simulink model "mariner_sim"  (R2018b)
(part 16 of 22)

  "IW{3,2}(6,:)'" : Constant  Value=[0.341232504422672555666196103629772551357746124267578125;-0.22407651602017242264963670095312409102916717529296875;-0.149532198205526156709055385363171808421611785888671875;-0.20169871649001336333384415411273948848247528076171875;0.1757399362782041396524590481931227259337902069091796875;0.05540417170915674927034189067853731103241443634033203125;0.0032609465010274645523080661035919547430239617824554443359375;-0.22300988569188906485152301684138365089893341064453125;-0.22795024991608858755398614448495209217071533203125;0.0919947464537682335627977181502501480281352996826171875;0.07236540787619029357902178389849723316729068756103515625;-0.019836013133734016478104678071758826263248920440673828125;-0.29188822221009502744237806837190873920917510986328125;0.30454637581194088369329620036296546459197998046875;-0.01535199508936785535440083805269750882871448993682861328125;0.36874333544784054783605142802116461098194122314453125;-0.361608618282780069908000086797983385622501373291015625;-0.30980629966419837018065663869492709636688232421875;-0.310442442961680609148089615700882859528064727783203125;0.006138782561133275007814180668219705694355070590972900390625;-0.1582495940895217445554266078033833764493465423583984375;-0.19808839258286281559406916130683384835720062255859375;0.0802930395519567408069150360461208038032054901123046875;-0.318214036272985889564068884283187799155712127685546875;0.0752733959769866789457637423765845596790313720703125;-0.34628170301207295000978092502919025719165802001953125;-0.09819346974937238903269332013223902322351932525634765625;0.221550156201519132803667844200390391051769256591796875;-0.1758804709099220098256211031184648163616657257080078125;-0.334406967215916950397769369374145753681659698486328125;-0.1193792720413492658426690695705474354326725006103515625;-0.1340589332285392620836006472018198110163211822509765625;-0.12205555886070197646464663421284058131277561187744140625;0.193328167325487909611325676451087929308414459228515625;0.247739557068020033181454664372722618281841278076171875;0.147170810348881853091285165646695531904697418212890625;0.2270252859387218713482781140555744059383869171142578125;-0.293548013190261858351703949665534310042858123779296875;0.2293318811175260041324008852825500071048736572265625;0.299951176935773056175804640588467009365558624267578125;-0.304346316698099972342106411815620958805084228515625;0.25577567358692754329041463279281742870807647705078125;-0.1015351339344442160861348156686290167272090911865234375;-0.134610152635351532079965863886172883212566375732421875;-0.11644572216746625070715737138016265816986560821533203125;-0.343208654547823233116332630743272602558135986328125;-0.11172239395568354936028043766782502643764019012451171875;0.0956567363935234282745767586675356142222881317138671875]
      mask Display: e = 0.06;c1 = [120 150 230]/255;c2 = ([120 150 230]+0)/383;c3 = ([120 150 230]+128)/383;patch([0 1 1 0],[0 0 1 1],c1);patch([0 1 1 1-e 1-e 0+e],[0 0 1 1-e 0+e 0+e],c2);patch([0 0 1 1-e 0+e 0+e],[0 1 1 1-e 1-e 0+e],c3);plot([0 1 1 0 0],[0 0 1 1 0]);disp('weights');
  "IW{3,2}(7,:)'" : Constant  Value=[-0.0848093278162808938969163818910601548850536346435546875;-0.00278975363091709706309107019706061691977083683013916015625;-0.09817238454077374665285304899953189305961132049560546875;0.228181011598485972147187794689671136438846588134765625;-0.00921754323048482558655702945316079421900212764739990234375;-0.04278287401801701694825652566578355617821216583251953125;-0.1989961874722619150634983498093788512051105499267578125;-0.18183822451057363167592484387569129467010498046875;0.2260092059368701000732215788957546465098857879638671875;-0.394935026337335182144983036778285168111324310302734375;-0.2167177061618534017473081121352151967585086822509765625;0.34819701323118390501321073315921239554882049560546875;0.1678517114742488214318427708349190652370452880859375;0.21633611008402819919638204737566411495208740234375;-0.279678431599733101631244380769203417003154754638671875;0.13924109951171226295940641648485325276851654052734375;0.04405273222892651385773632455311599187552928924560546875;-0.1635007783999306296696119034095318056643009185791015625;0.039552182620849307692623142429511062800884246826171875;-0.2712967951547629041897380375303328037261962890625;0.18092731846033316411848090865532867610454559326171875;0.2165878159643388756183668419907917268574237823486328125;0.15578599432246409417501809002715162932872772216796875;-0.1865871672175930806591992450194084085524082183837890625;0.139761063838464705266773080438724718987941741943359375;0.284453668022534522652478017334942705929279327392578125;-0.0240187759023694109850044497989074443466961383819580078125;0.23387180205340551975012886032345704734325408935546875;-0.335106083018000766582389360337401740252971649169921875;0.247786018469412672171614531180239282548427581787109375;-0.145089016439523266210898100325721316039562225341796875;0.31444505355689267300789424552931450307369232177734375;-0.195790615880808427373693803019705228507518768310546875;0.3180514946704551260125981571036390960216522216796875;-0.09295073257234624797273880858483607880771160125732421875;-0.315702391929300330009056096969288773834705352783203125;0.1299745945673785596508054140940657816827297210693359375;0.139781952709359280628831356807495467364788055419921875;-0.2260864659330905912515419231567648239433765411376953125;-0.30377892330009126364842586554004810750484466552734375;0.3620182776685598735610938092577271163463592529296875;-0.26409063788989473042789768442162312567234039306640625;0.033981677484790140386650136861135251820087432861328125;-0.10595438161818719613460615391886676661670207977294921875;0.323313510614337662474326862138696014881134033203125;0.1377493362885310601573252142770797945559024810791015625;0.1682723776856355490938454977367655374109745025634765625;-0.33705736528344465430251375437364913523197174072265625]
      mask Display: e = 0.06;c1 = [120 150 230]/255;c2 = ([120 150 230]+0)/383;c3 = ([120 150 230]+128)/383;patch([0 1 1 0],[0 0 1 1],c1);patch([0 1 1 1-e 1-e 0+e],[0 0 1 1-e 0+e 0+e],c2);patch([0 0 1 1-e 0+e 0+e],[0 1 1 1-e 1-e 0+e],c3);plot([0 1 1 0 0],[0 0 1 1 0]);disp('weights');
  "IW{3,2}(8,:)'" : Constant  Value=[0.039114358482732626554057020484833628870546817779541015625;0.1468831520343607810463737450845655985176563262939453125;0.2338793015886276027703871704943594522774219512939453125;-0.1284923546324590881706484424285008572041988372802734375;-0.2872511387092917534147318292525596916675567626953125;-0.03972391193774836570806741065098321996629238128662109375;-0.01429015337911259016234755137020329129882156848907470703125;0.172411094039722045945239869979559443891048431396484375;-0.321198867648277264219558446711744181811809539794921875;-0.11787302632761453846654831068008206784725189208984375;-0.05550699917852296161324687773230834864079952239990234375;-0.103636383004487020453865397939807735383510589599609375;-0.298020568488577219934398954137577675282955169677734375;0.14496903249883674735798422261723317205905914306640625;-0.326297358878205212562306769541464745998382568359375;-0.0301026617170235856468796242779717431403696537017822265625;0.21885743300318549753313845940283499658107757568359375;0.0249438383272913843935469913049018941819667816162109375;-0.291116601061845836628805272994213737547397613525390625;-0.348542440622258975491121191225829534232616424560546875;0.1149124389010942881572674423296120949089527130126953125;-0.302531514945001023253468019902356900274753570556640625;0.13508249841665931345602302826591767370700836181640625;0.1700053884746326737786858984691207297146320343017578125;-0.11814541620605405192190318075518007390201091766357421875;0.307383305246014426614920012070797383785247802734375;-0.151693805534957260050532568129710853099822998046875;-0.344792978103904967923654112382791936397552490234375;0.12067422165265494216068731248014955781400203704833984375;0.313131337233834183830794017922016791999340057373046875;-0.3218727309060369634607923217117786407470703125;0.122629299922777101894411089233472011983394622802734375;-0.11596149799633843902046947960116085596382617950439453125;-0.258397140883475484596232263356796465814113616943359375;-0.18391472175501999419822141135227866470813751220703125;-0.016084464502502483773671571043450967408716678619384765625;-0.31079529607058009599285242074984125792980194091796875;-0.166265953006079658660354425592231564223766326904296875;-0.352194230991786760842643388969008810818195343017578125;0.2426963474697447775696446115034632384777069091796875;-0.1805879178547815655520025757141411304473876953125;-0.267648024134625794889785765917622484266757965087890625;0.10022657443482944905621678799434448592364788055419921875;0.3075082791234569068450355189270339906215667724609375;0.17084270150574376589958092154120095074176788330078125;-0.337522936364130388131599147527595050632953643798828125;0.2126282074095191820806149962663766928017139434814453125;0.199427353419003139389786838364670984447002410888671875]
      mask Display: e = 0.06;c1 = [120 150 230]/255;c2 = ([120 150 230]+0)/383;c3 = ([120 150 230]+128)/383;patch([0 1 1 0],[0 0 1 1],c1);patch([0 1 1 1-e 1-e 0+e],[0 0 1 1-e 0+e 0+e],c2);patch([0 0 1 1-e 0+e 0+e],[0 1 1 1-e 1-e 0+e],c3);plot([0 1 1 0 0],[0 0 1 1 0]);disp('weights');
  "IW{3,2}(9,:)'" : Constant  Value=[-0.0238205677965650404470654422084407997317612171173095703125;0.243185697576507930950384661628049798309803009033203125;0.297800343945721690541716952793649397790431976318359375;0.360980778284137493461258827665005810558795928955078125;0.127393722859052538343149763022665865719318389892578125;-0.052279883862613306388933409607489011250436305999755859375;-0.2350807856437394927073825101615511812269687652587890625;-0.1691268633610674976264220958910300396382808685302734375;0.28876879465270210989302768211928196251392364501953125;-0.25464810083610112112495471592410467565059661865234375;-0.297217531797456524511602538041188381612300872802734375;-0.3531825895400888537523087506997399032115936279296875;0.29783631469964333415845203489880077540874481201171875;-0.2404837365605453636252519800109439529478549957275390625;0.25055933424268683751279240823350846767425537109375;-0.331121759202636034569167122754151932895183563232421875;-0.1939613285657608710010890717967413365840911865234375;-0.21222884241867479016008246617275290191173553466796875;-0.047235974253252703547456547994443099014461040496826171875;-0.08199746154330829484013776209394563920795917510986328125;-0.254206199542760191700807581582921557128429412841796875;0.1094792981275478638281128951348364353179931640625;-0.221805794568943337452537889475934207439422607421875;0.08105592581627256432152961451720329932868480682373046875;0.08153776128372525189291764036170206964015960693359375;-0.12418834564838605871717192030700971372425556182861328125;0.317661897582970198516960635970463044941425323486328125;0.279103037699123424086877776062465272843837738037109375;-0.0314143521071133247080098271908354945480823516845703125;-0.0277297961896677651327802749392503756098449230194091796875;0.0094918260980598433140809078167876577936112880706787109375;-0.113651149579278409884608436186681501567363739013671875;-0.235044333000665961463937492226250469684600830078125;-0.020301442888306188427893772541210637427866458892822265625;-0.205062843425597607360799656817107461392879486083984375;-0.355762679220968436322181105424533598124980926513671875;-0.318004263198188474870420350271160714328289031982421875;0.09913056476287489260368346322138677351176738739013671875;0.2461888821106313629538675513686030171811580657958984375;-0.29662946668134793082316491563688032329082489013671875;-0.303087653528123002200089786128955893218517303466796875;0.118432781086760863242801633532508276402950286865234375;-0.15430646723824714694472959308768622577190399169921875;0.333492763836934880128382019393029622733592987060546875;-0.1494036524887753791812627923718537203967571258544921875;-0.2116953685190388345649381562907365150749683380126953125;-0.0958569890792293488601671924698166549205780029296875;0.0239658688517560940212103304247648338787257671356201171875]
      mask Display: e = 0.06;c1 = [120 150 230]/255;c2 = ([120 150 230]+0)/383;c3 = ([120 150 230]+128)/383;patch([0 1 1 0],[0 0 1 1],c1);patch([0 1 1 1-e 1-e 0+e],[0 0 1 1-e 0+e 0+e],c2);patch([0 0 1 1-e 0+e 0+e],[0 1 1 1-e 1-e 0+e],c3);plot([0 1 1 0 0],[0 0 1 1 0]);disp('weights');
  Mux : Mux  Inputs=48
      mask Display: e = 0.06;c1 = [120 150 230]/255;c2 = ([120 150 230]+0)/383;c3 = ([120 150 230]+128)/383;patch([0 1 1 0],[0 0 1 1],c1);patch([0 1 1 1-e 1-e 0+e],[0 0 1 1-e 0+e 0+e],c2);patch([0 0 1 1-e 0+e 0+e],[0 1 1 1-e 1-e 0+e],c3);plot([0 1 1 0 0],[0 0 1 1 0]);disp('Mux');
  dotprod{1..48} (48 alike) : neural/Weight Functions/dotprod
  "lz{3,2}" : Outport
      mask Display: e = 0.06;c1 = [120 230 180]/255;c2 = ([120 230 180]+0)/(256+128);c3 = ([120 230 180]+128)/(256+128);patch([0 1 1 0],[0 0 1 1],c1);patch([0 1 1 1-e 1-e 0+e],[0 0 1 1-e 0+e 0+e],c2);patch([0 0 1 1-e 0+e 0+e],[0 1 1 1-e 1-e 0+e],c3);plot([0 1 1 0 0],[0 0 1 1 0]);
  wires:
  Mux/1 -> "lz{3,2}"/1
  dotprod48/1 -> Mux/48
  "IW{3,2}(48,:)'"/1 -> dotprod48/1
  dotprod47/1 -> Mux/47
  "IW{3,2}(47,:)'"/1 -> dotprod47/1
  dotprod46/1 -> Mux/46
  "IW{3,2}(46,:)'"/1 -> dotprod46/1
  dotprod45/1 -> Mux/45
  "IW{3,2}(45,:)'"/1 -> dotprod45/1
  dotprod44/1 -> Mux/44
  "IW{3,2}(44,:)'"/1 -> dotprod44/1
  dotprod43/1 -> Mux/43
  "IW{3,2}(43,:)'"/1 -> dotprod43/1
  dotprod42/1 -> Mux/42
  "IW{3,2}(42,:)'"/1 -> dotprod42/1
  dotprod41/1 -> Mux/41
  "IW{3,2}(41,:)'"/1 -> dotprod41/1
  dotprod40/1 -> Mux/40
  "IW{3,2}(40,:)'"/1 -> dotprod40/1
  dotprod39/1 -> Mux/39
  "IW{3,2}(39,:)'"/1 -> dotprod39/1
  dotprod38/1 -> Mux/38
  "IW{3,2}(38,:)'"/1 -> dotprod38/1
  dotprod37/1 -> Mux/37
  "IW{3,2}(37,:)'"/1 -> dotprod37/1
  dotprod36/1 -> Mux/36
  "IW{3,2}(36,:)'"/1 -> dotprod36/1
  dotprod35/1 -> Mux/35
  "IW{3,2}(35,:)'"/1 -> dotprod35/1
  dotprod34/1 -> Mux/34
  "IW{3,2}(34,:)'"/1 -> dotprod34/1
  dotprod33/1 -> Mux/33
  "IW{3,2}(33,:)'"/1 -> dotprod33/1
  dotprod32/1 -> Mux/32
  "IW{3,2}(32,:)'"/1 -> dotprod32/1
  dotprod31/1 -> Mux/31
  "IW{3,2}(31,:)'"/1 -> dotprod31/1
  dotprod30/1 -> Mux/30
  "IW{3,2}(30,:)'"/1 -> dotprod30/1
  dotprod29/1 -> Mux/29
  "IW{3,2}(29,:)'"/1 -> dotprod29/1
  dotprod28/1 -> Mux/28
  "IW{3,2}(28,:)'"/1 -> dotprod28/1
  dotprod27/1 -> Mux/27
  "IW{3,2}(27,:)'"/1 -> dotprod27/1
  dotprod26/1 -> Mux/26
  "IW{3,2}(26,:)'"/1 -> dotprod26/1
  dotprod25/1 -> Mux/25
  "IW{3,2}(25,:)'"/1 -> dotprod25/1
  dotprod24/1 -> Mux/24
  "IW{3,2}(24,:)'"/1 -> dotprod24/1
  dotprod23/1 -> Mux/23
  "IW{3,2}(23,:)'"/1 -> dotprod23/1
  dotprod22/1 -> Mux/22
  "IW{3,2}(22,:)'"/1 -> dotprod22/1
  dotprod21/1 -> Mux/21
  "IW{3,2}(21,:)'"/1 -> dotprod21/1
  dotprod20/1 -> Mux/20
  "IW{3,2}(20,:)'"/1 -> dotprod20/1
  dotprod19/1 -> Mux/19
  "IW{3,2}(19,:)'"/1 -> dotprod19/1
  dotprod18/1 -> Mux/18
  "IW{3,2}(18,:)'"/1 -> dotprod18/1
  dotprod17/1 -> Mux/17
  "IW{3,2}(17,:)'"/1 -> dotprod17/1
  dotprod16/1 -> Mux/16
  "IW{3,2}(16,:)'"/1 -> dotprod16/1
  dotprod15/1 -> Mux/15
  "IW{3,2}(15,:)'"/1 -> dotprod15/1
  dotprod14/1 -> Mux/14
  "IW{3,2}(14,:)'"/1 -> dotprod14/1
  dotprod13/1 -> Mux/13
  "IW{3,2}(13,:)'"/1 -> dotprod13/1
  dotprod12/1 -> Mux/12
  "IW{3,2}(12,:)'"/1 -> dotprod12/1
  dotprod11/1 -> Mux/11
  "IW{3,2}(11,:)'"/1 -> dotprod11/1
  dotprod10/1 -> Mux/10
  "IW{3,2}(10,:)'"/1 -> dotprod10/1
  dotprod9/1 -> Mux/9
  "IW{3,2}(9,:)'"/1 -> dotprod9/1
  dotprod8/1 -> Mux/8
  "IW{3,2}(8,:)'"/1 -> dotprod8/1
  dotprod7/1 -> Mux/7
  "IW{3,2}(7,:)'"/1 -> dotprod7/1
  dotprod6/1 -> Mux/6
  "IW{3,2}(6,:)'"/1 -> dotprod6/1
  dotprod5/1 -> Mux/5
  "IW{3,2}(5,:)'"/1 -> dotprod5/1
  dotprod4/1 -> Mux/4
  "IW{3,2}(4,:)'"/1 -> dotprod4/1
  dotprod3/1 -> Mux/3
  "IW{3,2}(3,:)'"/1 -> dotprod3/1
  dotprod2/1 -> Mux/2
  "IW{3,2}(2,:)'"/1 -> dotprod2/1
  dotprod1/1 -> Mux/1
  "ad{3,2}"/1 -> dotprod48/2, dotprod47/2, dotprod46/2, dotprod45/2, dotprod44/2, dotprod43/2, dotprod42/2, dotprod41/2, dotprod40/2, dotprod39/2, dotprod38/2, dotprod37/2, dotprod36/2, dotprod35/2, dotprod34/2, dotprod33/2, dotprod32/2, dotprod31/2, dotprod30/2, dotprod29/2, dotprod28/2, dotprod27/2, dotprod26/2, dotprod25/2, dotprod24/2, dotprod23/2, dotprod22/2, dotprod21/2, dotprod20/2, dotprod19/2, dotprod18/2, dotprod17/2, dotprod16/2, dotprod15/2, dotprod14/2, dotprod13/2, dotprod12/2, dotprod11/2, dotprod10/2, dotprod9/2, dotprod8/2, dotprod7/2, dotprod6/2, dotprod5/2, dotprod4/2, dotprod3/2, dotprod2/2, dotprod1/2
  "IW{3,2}(1,:)'"/1 -> dotprod1/1
